simulink model "martin_arbot_v2offset"  (R2020a)
settings: Solver=ode15s  StartTime=0.0  StopTime=15  MaxStep=.01  RelTol=1e-3  AbsTol=1e-4
InitFcn:
  | % currentFolder = pwd;
  | % parent = '../Targeting';
  | % environment = '../Environment';
  | % addpath(genpath(parent));
  | % addpath(genpath(environment));
  | 
  | startup_ARbot;
  | chute2_DataFile;
  | guard_DataFile1;
  | shelf_DataFile1;
  | bin_assembly_DataFile;
values from neighbouring files (symbols this model uses):
  Environment = append(cwd,'/Environment')    [init_root_paths_mac.m]    (also in init_root_paths_windows.m = append(cwd,'\Environment'))
undefined symbols (not defined in the file or in its folder): belt_h, belt_l, belt_spd, belt_w, box1_dim, box2_dim, box3_dim, box4_dim, box5_dim, cube_d, deposit_joint_angle, Extr_Data_LinkHoles, floor_d, floor_l, ikSol, initial_joints, m, n, P_C, safe_via_angles, sigbuilder_block, smiData, X, Y, Z
libraries: sm_lib x145, nesl_utility x78, Contact_Forces_Lib x10, simulink x5, Parts_Lib x5, dspsrcs4 x1
(part 4 of 5)

== system martin_arbot_v2offset/Bin//guard//shelf1/guard_1_RIGID2 ==
  ReferenceFrame : sm_lib/Frames and Transforms/Reference Frame
  Solid : sm_lib/Body Elements/File Solid  ExtGeomFileName=/Users/mcontr/repos/ARbot_Simulink/v3/Environment/meshes/guard_Default_sldprt.STEP  UnitType=FromFile  ExtGeomFileUnits=m  StepReaderType=HEX  ExportConvexHullGeometry=off  InertiaType=Custom  Mass=smiData.Solid(1).mass  MassUnits=kg  CenterOfMass=smiData.Solid(1).CoM  CenterOfMassUnits=in  MomentsOfInertia=smiData.Solid(1).MoI  MomentsOfInertiaUnits=kg*in^2  ProductsOfInertia=smiData.Solid(1).PoI  ProductsOfInertiaUnits=kg*in^2  BasedOnType=DensityFromFile  Density=1000  DensityUnits=kg/m^3  DoExposeReferenceFrame=on  SerializedFrames=<Frames/>  GraphicType=FromGeometry  MarkerShape=Sphere  MarkerSize=10  GraphicVisPropType=SimpleVisualProperties  GraphicDiffuseColor=smiData.Solid(1).color  GraphicSpecularColor=[0.5 0.5 0.5 1.0]  GraphicAmbientColor=[0.15 0.15 0.15 1.0]  GraphicEmissiveColor=[0.0 0.0 0.0 1.0]  GraphicShininess=75  GraphicOpacity=smiData.Solid(1).opacity
  F : PMIOPort  Side=Left
  connections:
  ReferenceFrame/RConn1 -- Solid/RConn1 -- F/RConn1

== system martin_arbot_v2offset/Bin//guard//shelf1/guard_1_RIGID3 ==
  ReferenceFrame : sm_lib/Frames and Transforms/Reference Frame
  Solid : sm_lib/Body Elements/File Solid  ExtGeomFileName=/Users/mcontr/repos/ARbot_Simulink/v3/Environment/meshes/guard_Default_sldprt.STEP  UnitType=FromFile  ExtGeomFileUnits=m  StepReaderType=HEX  ExportConvexHullGeometry=off  InertiaType=Custom  Mass=smiData.Solid(1).mass  MassUnits=kg  CenterOfMass=smiData.Solid(1).CoM  CenterOfMassUnits=in  MomentsOfInertia=smiData.Solid(1).MoI  MomentsOfInertiaUnits=kg*in^2  ProductsOfInertia=smiData.Solid(1).PoI  ProductsOfInertiaUnits=kg*in^2  BasedOnType=DensityFromFile  Density=1000  DensityUnits=kg/m^3  DoExposeReferenceFrame=on  SerializedFrames=<Frames/>  GraphicType=FromGeometry  MarkerShape=Sphere  MarkerSize=10  GraphicVisPropType=SimpleVisualProperties  GraphicDiffuseColor=smiData.Solid(1).color  GraphicSpecularColor=[0.5 0.5 0.5 1.0]  GraphicAmbientColor=[0.15 0.15 0.15 1.0]  GraphicEmissiveColor=[0.0 0.0 0.0 1.0]  GraphicShininess=75  GraphicOpacity=smiData.Solid(1).opacity
  F : PMIOPort  Side=Left
  connections:
  ReferenceFrame/RConn1 -- Solid/RConn1 -- F/RConn1

== system martin_arbot_v2offset/Bin//guard//shelf1/shelf_1_RIGID1 ==
  ReferenceFrame : sm_lib/Frames and Transforms/Reference Frame
  Solid : sm_lib/Body Elements/File Solid  ExtGeomFileName=/Users/mcontr/repos/ARbot_Simulink/v3/Environment/meshes/shelf_Default_sldprt.STEP  UnitType=FromFile  ExtGeomFileUnits=m  StepReaderType=HEX  ExportConvexHullGeometry=off  InertiaType=Custom  Mass=smiData.Solid(1).mass  MassUnits=kg  CenterOfMass=smiData.Solid(1).CoM  CenterOfMassUnits=in  MomentsOfInertia=smiData.Solid(1).MoI  MomentsOfInertiaUnits=kg*in^2  ProductsOfInertia=smiData.Solid(1).PoI  ProductsOfInertiaUnits=kg*in^2  BasedOnType=DensityFromFile  Density=1000  DensityUnits=kg/m^3  DoExposeReferenceFrame=on  SerializedFrames=<Frames/>  GraphicType=FromGeometry  MarkerShape=Sphere  MarkerSize=10  GraphicVisPropType=SimpleVisualProperties  GraphicDiffuseColor=smiData.Solid(1).color  GraphicSpecularColor=[0.5 0.5 0.5 1.0]  GraphicAmbientColor=[0.15 0.15 0.15 1.0]  GraphicEmissiveColor=[0.0 0.0 0.0 1.0]  GraphicShininess=75  GraphicOpacity=smiData.Solid(1).opacity
  F : PMIOPort  Side=Left
  connections:
  ReferenceFrame/RConn1 -- Solid/RConn1 -- F/RConn1

== system martin_arbot_v2offset/Box1/Box1 ==
  Box : sm_lib/Body Elements/Brick Solid  GraphicAmbientColor=[0.15 0.15 0.15 1.0]  BasedOnType=Density  BrickDimensions=box1_dim  BrickDimensionUnits=m  CenterOfMass=[0 0 0]  CenterOfMassUnits=m  GraphicDiffuseColor=[0.7 0.3 .08]  Density=1000  DensityUnits=kg/m^3  DoExposeReferenceFrame=on  GraphicEmissiveColor=[0.0 0.0 0.0 1.0]  ExportEntireGeometry=off  SerializedFrames=<Frames/>  MarkerShape=Sphere  MarkerSize=10  GraphicType=FromGeometry  InertiaType=CalculateFromGeometry  Mass=1  MassUnits=kg  MomentsOfInertia=[1 1 1]  MomentsOfInertiaUnits=kg*m^2  GraphicOpacity=1.0  ProductsOfInertia=[1 1 1]  ProductsOfInertiaUnits=kg*m^2  GraphicShininess=75  GraphicSpecularColor=[0.5 0.5 0.5 1.0]  GraphicVisPropType=SimpleVisualProperties
  Transform Face px : sm_lib/Frames and Transforms/Rigid Transform  TranslationMethod=Cartesian  TranslationStandardOffset=0  TranslationLengthUnit=m  TranslationStandardAxis=+Z  TranslationCartesianOffset=[0 0 -box1_dim(3)*.5]  TranslationROffset=0  TranslationROffsetUnits=m  TranslationZOffset=0  TranslationZOffsetUnits=m  TranslationThetaOffset=0  TranslationThetaOffsetUnits=deg  RotationMethod=StandardAxis  RotationAngleUnits=deg  RotationStandardAxis=+X  RotationAngle=-180  RotationArbitraryAxis=[0 0 1]  FollAlignAxisA=+X  BaseAlignAxisA=+Y  FollAlignAxisB=+Y  BaseAlignAxisB=+Z  RotationSequenceAxes=FollowerAxes  RotationSequence=XYX  RotationSequenceAngles=[0 0 0]  RotationSequenceAnglesUnits=deg  RotationMatrix=[1 0 0; 0 1 0; 0 0 1]
  Fa : PMIOPort  Side=Right
  F : PMIOPort  Port=2  Side=Left
  connections:
  Fa/RConn1 -- Transform Face px/RConn1
  Transform Face px/LConn1 -- F/RConn1 -- Box/RConn1

== system martin_arbot_v2offset/Box1/Create Bus Belt In5 ==
  On : Inport
  Belt Speed : Gain  Gain=belt_spd
  Bus Creator : BusCreator  Inputs=3
  Constant : Constant
  Constant1 : Constant  Value=0
  bus : Outport  VectorParamsAs1DForOutWhenUnconnected=off
  wires:
  Constant1/1 -> Bus Creator/3  "vy"
  On/1 -> Belt Speed/1
  Constant/1 -> Bus Creator/1  "Enable"
  Bus Creator/1 -> bus/1
  Belt Speed/1 -> Bus Creator/2  "vx"

== system martin_arbot_v2offset/Box1/Forces5 ==
  B1 : Inport
  Bus Selector : BusSelector  OutputSignals=fz1.Normal Force,fz2.Normal Force,fz3.Normal Force,fz4.Normal Force
  Mux : Mux
  Fn1 : Outport  VectorParamsAs1DForOutWhenUnconnected=off
  wires:
  B1/1 -> Bus Selector/1
  Bus Selector/3 -> Mux/3  "<Normal Force>"
  Bus Selector/4 -> Mux/4  "<Normal Force>"
  Bus Selector/2 -> Mux/2  "<Normal Force>"
  Bus Selector/1 -> Mux/1  "<Normal Force>"
  Mux/1 -> Fn1/1

== system martin_arbot_v2offset/Box2/Box2 ==
  Box : sm_lib/Body Elements/Brick Solid  GraphicAmbientColor=[0.15 0.15 0.15 1.0]  BasedOnType=Density  BrickDimensions=box2_dim  BrickDimensionUnits=m  CenterOfMass=[0 0 0]  CenterOfMassUnits=m  GraphicDiffuseColor=[0.4 0.2 0.3]  Density=1000  DensityUnits=kg/m^3  DoExposeReferenceFrame=on  GraphicEmissiveColor=[0.0 0.0 0.0 1.0]  ExportEntireGeometry=off  SerializedFrames=<Frames/>  MarkerShape=Sphere  MarkerSize=10  GraphicType=FromGeometry  InertiaType=CalculateFromGeometry  Mass=1  MassUnits=kg  MomentsOfInertia=[1 1 1]  MomentsOfInertiaUnits=kg*m^2  GraphicOpacity=1.0  ProductsOfInertia=[1 1 1]  ProductsOfInertiaUnits=kg*m^2  GraphicShininess=75  GraphicSpecularColor=[0.5 0.5 0.5 1.0]  GraphicVisPropType=SimpleVisualProperties
  Transform Face px : sm_lib/Frames and Transforms/Rigid Transform  TranslationMethod=Cartesian  TranslationStandardOffset=0  TranslationLengthUnit=m  TranslationStandardAxis=+Z  TranslationCartesianOffset=[0 0 -box2_dim(3)*.5]  TranslationROffset=0  TranslationROffsetUnits=m  TranslationZOffset=0  TranslationZOffsetUnits=m  TranslationThetaOffset=0  TranslationThetaOffsetUnits=deg  RotationMethod=StandardAxis  RotationAngleUnits=deg  RotationStandardAxis=+X  RotationAngle=-180  RotationArbitraryAxis=[0 0 1]  FollAlignAxisA=+X  BaseAlignAxisA=+Y  FollAlignAxisB=+Y  BaseAlignAxisB=+Z  RotationSequenceAxes=FollowerAxes  RotationSequence=XYX  RotationSequenceAngles=[0 0 0]  RotationSequenceAnglesUnits=deg  RotationMatrix=[1 0 0; 0 1 0; 0 0 1]
  Fa : PMIOPort  Side=Right
  F : PMIOPort  Port=2  Side=Left
  connections:
  Fa/RConn1 -- Transform Face px/RConn1
  Transform Face px/LConn1 -- F/RConn1 -- Box/RConn1

== system martin_arbot_v2offset/Box2/Create Bus Belt In4 ==
  On : Inport
  Belt Speed : Gain  Gain=belt_spd
  Bus Creator : BusCreator  Inputs=3
  Constant : Constant
  Constant1 : Constant  Value=0
  bus : Outport  VectorParamsAs1DForOutWhenUnconnected=off
  wires:
  Constant1/1 -> Bus Creator/3  "vy"
  On/1 -> Belt Speed/1
  Constant/1 -> Bus Creator/1  "Enable"
  Bus Creator/1 -> bus/1
  Belt Speed/1 -> Bus Creator/2  "vx"

== system martin_arbot_v2offset/Box2/Forces4 ==
  B1 : Inport
  Bus Selector : BusSelector  OutputSignals=fz1.Normal Force,fz2.Normal Force,fz3.Normal Force,fz4.Normal Force
  Mux : Mux
  Fn1 : Outport  VectorParamsAs1DForOutWhenUnconnected=off
  wires:
  B1/1 -> Bus Selector/1
  Bus Selector/3 -> Mux/3  "<Normal Force>"
  Bus Selector/4 -> Mux/4  "<Normal Force>"
  Bus Selector/2 -> Mux/2  "<Normal Force>"
  Bus Selector/1 -> Mux/1  "<Normal Force>"
  Mux/1 -> Fn1/1

== system martin_arbot_v2offset/Box3/Box3 ==
  Box : sm_lib/Body Elements/Brick Solid  GraphicAmbientColor=[0.15 0.15 0.15 1.0]  BasedOnType=Density  BrickDimensions=box3_dim  BrickDimensionUnits=m  CenterOfMass=[0 0 0]  CenterOfMassUnits=m  GraphicDiffuseColor=[0.2 0.2 1.0]  Density=1000  DensityUnits=kg/m^3  DoExposeReferenceFrame=on  GraphicEmissiveColor=[0.0 0.0 0.0 1.0]  ExportEntireGeometry=off  SerializedFrames=<Frames/>  MarkerShape=Sphere  MarkerSize=10  GraphicType=FromGeometry  InertiaType=CalculateFromGeometry  Mass=1  MassUnits=kg  MomentsOfInertia=[1 1 1]  MomentsOfInertiaUnits=kg*m^2  GraphicOpacity=1.0  ProductsOfInertia=[1 1 1]  ProductsOfInertiaUnits=kg*m^2  GraphicShininess=75  GraphicSpecularColor=[0.5 0.5 0.5 1.0]  GraphicVisPropType=SimpleVisualProperties
  Transform Face px : sm_lib/Frames and Transforms/Rigid Transform  TranslationMethod=Cartesian  TranslationStandardOffset=0  TranslationLengthUnit=m  TranslationStandardAxis=+Z  TranslationCartesianOffset=[0 0 -box3_dim(3)*.5]  TranslationROffset=0  TranslationROffsetUnits=m  TranslationZOffset=0  TranslationZOffsetUnits=m  TranslationThetaOffset=0  TranslationThetaOffsetUnits=deg  RotationMethod=StandardAxis  RotationAngleUnits=deg  RotationStandardAxis=+X  RotationAngle=-180  RotationArbitraryAxis=[0 0 1]  FollAlignAxisA=+X  BaseAlignAxisA=+Y  FollAlignAxisB=+Y  BaseAlignAxisB=+Z  RotationSequenceAxes=FollowerAxes  RotationSequence=XYX  RotationSequenceAngles=[0 0 0]  RotationSequenceAnglesUnits=deg  RotationMatrix=[1 0 0; 0 1 0; 0 0 1]
  Fa : PMIOPort  Side=Right
  F : PMIOPort  Port=2  Side=Left
  connections:
  Fa/RConn1 -- Transform Face px/RConn1
  Transform Face px/LConn1 -- F/RConn1 -- Box/RConn1

== system martin_arbot_v2offset/Box3/Create Bus Belt In3 ==
  On : Inport
  Belt Speed : Gain  Gain=belt_spd
  Bus Creator : BusCreator  Inputs=3
  Constant : Constant
  Constant1 : Constant  Value=0
  bus : Outport  VectorParamsAs1DForOutWhenUnconnected=off
  wires:
  Constant1/1 -> Bus Creator/3  "vy"
  On/1 -> Belt Speed/1
  Constant/1 -> Bus Creator/1  "Enable"
  Bus Creator/1 -> bus/1
  Belt Speed/1 -> Bus Creator/2  "vx"

== system martin_arbot_v2offset/Box3/Forces3 ==
  B1 : Inport
  Bus Selector : BusSelector  OutputSignals=fz1.Normal Force,fz2.Normal Force,fz3.Normal Force,fz4.Normal Force
  Mux : Mux
  Fn1 : Outport  VectorParamsAs1DForOutWhenUnconnected=off
  wires:
  B1/1 -> Bus Selector/1
  Bus Selector/3 -> Mux/3  "<Normal Force>"
  Bus Selector/4 -> Mux/4  "<Normal Force>"
  Bus Selector/2 -> Mux/2  "<Normal Force>"
  Bus Selector/1 -> Mux/1  "<Normal Force>"
  Mux/1 -> Fn1/1

== system martin_arbot_v2offset/Box4/Box4 ==
  Box : sm_lib/Body Elements/Brick Solid  GraphicAmbientColor=[0.15 0.15 0.15 1.0]  BasedOnType=Density  BrickDimensions=box4_dim  BrickDimensionUnits=m  CenterOfMass=[0 0 0]  CenterOfMassUnits=m  GraphicDiffuseColor=[0.4 0.8 0.2]  Density=1000  DensityUnits=kg/m^3  DoExposeReferenceFrame=on  GraphicEmissiveColor=[0.0 0.0 0.0 1.0]  ExportEntireGeometry=off  SerializedFrames=<Frames/>  MarkerShape=Sphere  MarkerSize=10  GraphicType=FromGeometry  InertiaType=CalculateFromGeometry  Mass=1  MassUnits=kg  MomentsOfInertia=[1 1 1]  MomentsOfInertiaUnits=kg*m^2  GraphicOpacity=1.0  ProductsOfInertia=[1 1 1]  ProductsOfInertiaUnits=kg*m^2  GraphicShininess=75  GraphicSpecularColor=[0.5 0.5 0.5 1.0]  GraphicVisPropType=SimpleVisualProperties
  Transform Face px : sm_lib/Frames and Transforms/Rigid Transform  TranslationMethod=Cartesian  TranslationStandardOffset=0  TranslationLengthUnit=m  TranslationStandardAxis=+Z  TranslationCartesianOffset=[0 0 -box4_dim(3)*.5]  TranslationROffset=0  TranslationROffsetUnits=m  TranslationZOffset=0  TranslationZOffsetUnits=m  TranslationThetaOffset=0  TranslationThetaOffsetUnits=deg  RotationMethod=StandardAxis  RotationAngleUnits=deg  RotationStandardAxis=+X  RotationAngle=-180  RotationArbitraryAxis=[0 0 1]  FollAlignAxisA=+X  BaseAlignAxisA=+Y  FollAlignAxisB=+Y  BaseAlignAxisB=+Z  RotationSequenceAxes=FollowerAxes  RotationSequence=XYX  RotationSequenceAngles=[0 0 0]  RotationSequenceAnglesUnits=deg  RotationMatrix=[1 0 0; 0 1 0; 0 0 1]
  Fa : PMIOPort  Side=Right
  F : PMIOPort  Port=2  Side=Left
  connections:
  Fa/RConn1 -- Transform Face px/RConn1
  Transform Face px/LConn1 -- F/RConn1 -- Box/RConn1

== system martin_arbot_v2offset/Box4/Create Bus Belt In1 ==
  On : Inport
  Belt Speed : Gain  Gain=belt_spd
  Bus Creator : BusCreator  Inputs=3
  Constant : Constant
  Constant1 : Constant  Value=0
  bus : Outport  VectorParamsAs1DForOutWhenUnconnected=off
  wires:
  Constant1/1 -> Bus Creator/3  "vy"
  On/1 -> Belt Speed/1
  Constant/1 -> Bus Creator/1  "Enable"
  Bus Creator/1 -> bus/1
  Belt Speed/1 -> Bus Creator/2  "vx"

== system martin_arbot_v2offset/Box4/Forces1 ==
  B1 : Inport
  Bus Selector : BusSelector  OutputSignals=fz1.Normal Force,fz2.Normal Force,fz3.Normal Force,fz4.Normal Force
  Mux : Mux
  Fn1 : Outport  VectorParamsAs1DForOutWhenUnconnected=off
  wires:
  B1/1 -> Bus Selector/1
  Bus Selector/3 -> Mux/3  "<Normal Force>"
  Bus Selector/4 -> Mux/4  "<Normal Force>"
  Bus Selector/2 -> Mux/2  "<Normal Force>"
  Bus Selector/1 -> Mux/1  "<Normal Force>"
  Mux/1 -> Fn1/1

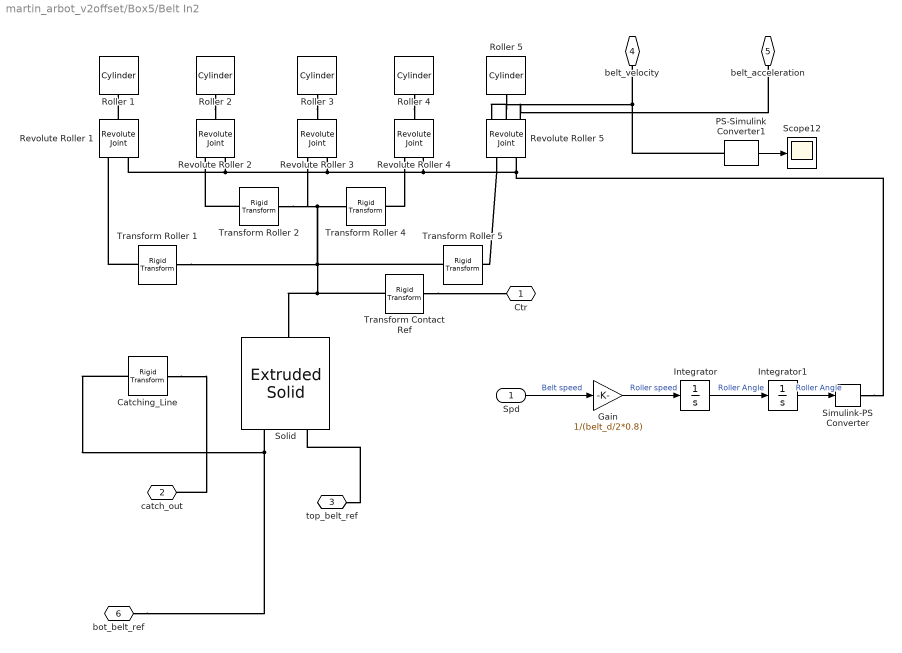
== system martin_arbot_v2offset/Box5/Belt In2 ==
  Spd : Inport
  Catching_Line : sm_lib/Frames and Transforms/Rigid Transform  TranslationMethod=StandardAxis  TranslationStandardOffset=catch_line_dist  TranslationLengthUnit=m  TranslationStandardAxis=+Y  TranslationCartesianOffset=[0 0 0]  TranslationROffset=0  TranslationROffsetUnits=m  TranslationZOffset=0  TranslationZOffsetUnits=m  TranslationThetaOffset=0  TranslationThetaOffsetUnits=deg  RotationMethod=StandardAxis  RotationAngleUnits=deg  RotationStandardAxis=+Y  RotationAngle=0.0  RotationArbitraryAxis=[0 0 1]  FollAlignAxisA=+X  BaseAlignAxisA=+Y  FollAlignAxisB=+Y  BaseAlignAxisB=+Z  RotationSequenceAxes=FollowerAxes  RotationSequence=XYX  RotationSequenceAngles=[0 0 0]  RotationSequenceAnglesUnits=deg  RotationMatrix=[1 0 0; 0 1 0; 0 0 1]
  Gain : Gain  Gain=1/(belt_d/2*0.8)
  Integrator : Integrator  InitialCondition=12.5049999999999
  Integrator1 : Integrator  InitialCondition=12.5049999999999
  PS-Simulink Converter1 : nesl_utility/PS-Simulink Converter  PhysicalDomain=network_engine_domain  SubClassName=ps_output  LeftPortType=input  RightPortType=output  PseudoPeriodic=off  Frequencies=[]  Unit=inherit  AffineConversion=off
  Revolute Roller {1..4} (4 alike) : sm_lib/Joints/Revolute Joint  JointMode=Normal  SenseConstraintForce=off  SenseConstraintForceX=off  SenseConstraintForceY=off  SenseConstraintForceZ=off  SenseConstraintTorque=off  SenseConstraintTorqueX=off  SenseConstraintTorqueY=off  SenseConstraintTorqueZ=off  SenseTotalForce=off  SenseTotalForceX=off  SenseTotalForceY=off  SenseTotalForceZ=off  SenseTotalTorque=off  SenseTotalTorqueX=off  SenseTotalTorqueY=off  SenseTotalTorqueZ=off  CompositeWrenchDir=FollowerOnBase  CompositeWrenchFrame=BaseFrame  EquilibriumPosition=0  EquilibriumPositionUnits=deg  SpringStiffness=0  SpringStiffnessUnits=N*m/deg  DampingCoefficient=0  DampingCoefficientUnits=N*m/(deg/s)  TorqueActuationMode=ComputedTorque  MotionActuationMode=InputMotion  SensePosition=off  SenseVelocity=off  SenseAcceleration=off  SenseTorqueForce=off  SenseLowerLimitTorqueForce=off  SenseUpperLimitTorqueForce=off  LowerLimitSpecify=off  LowerLimitBound=-90  LowerLimitBoundUnits=deg  LowerLimitStiffness=1e4  LowerLimitStiffnessUnits=N*m/deg  LowerLimitDamping=10  LowerLimitDampingUnits=N*m/(deg/s)  LowerLimitTransitionRegionWidth=0.1  LowerLimitTransitionRegionWidthUnits=deg  UpperLimitSpecify=off  UpperLimitBound=90  UpperLimitBoundUnits=deg  UpperLimitStiffness=1e4  UpperLimitStiffnessUnits=N*m/deg  UpperLimitDamping=10  UpperLimitDampingUnits=N*m/(deg/s)  UpperLimitTransitionRegionWidth=0.1  UpperLimitTransitionRegionWidthUnits=deg  PositionTargetSpecify=off  PositionTargetPriority=High  PositionTargetValue=0  PositionTargetValueUnits=deg  VelocityTargetSpecify=on  VelocityTargetPriority=High  VelocityTargetValue=12.5049999999992  VelocityTargetValueUnits=deg/s
  Revolute Roller 5 : sm_lib/Joints/Revolute Joint  JointMode=Normal  SenseConstraintForce=off  SenseConstraintForceX=off  SenseConstraintForceY=off  SenseConstraintForceZ=off  SenseConstraintTorque=off  SenseConstraintTorqueX=off  SenseConstraintTorqueY=off  SenseConstraintTorqueZ=off  SenseTotalForce=off  SenseTotalForceX=off  SenseTotalForceY=off  SenseTotalForceZ=off  SenseTotalTorque=off  SenseTotalTorqueX=off  SenseTotalTorqueY=off  SenseTotalTorqueZ=off  CompositeWrenchDir=FollowerOnBase  CompositeWrenchFrame=BaseFrame  EquilibriumPosition=0  EquilibriumPositionUnits=deg  SpringStiffness=0  SpringStiffnessUnits=N*m/deg  DampingCoefficient=0  DampingCoefficientUnits=N*m/(deg/s)  TorqueActuationMode=ComputedTorque  MotionActuationMode=InputMotion  SensePosition=off  SenseVelocity=on  SenseAcceleration=on  SenseTorqueForce=off  SenseLowerLimitTorqueForce=off  SenseUpperLimitTorqueForce=off  LowerLimitSpecify=off  LowerLimitBound=-90  LowerLimitBoundUnits=deg  LowerLimitStiffness=1e4  LowerLimitStiffnessUnits=N*m/deg  LowerLimitDamping=10  LowerLimitDampingUnits=N*m/(deg/s)  LowerLimitTransitionRegionWidth=0.1  LowerLimitTransitionRegionWidthUnits=deg  UpperLimitSpecify=off  UpperLimitBound=90  UpperLimitBoundUnits=deg  UpperLimitStiffness=1e4  UpperLimitStiffnessUnits=N*m/deg  UpperLimitDamping=10  UpperLimitDampingUnits=N*m/(deg/s)  UpperLimitTransitionRegionWidth=0.1  UpperLimitTransitionRegionWidthUnits=deg  PositionTargetSpecify=off  PositionTargetPriority=High  PositionTargetValue=0  PositionTargetValueUnits=deg  VelocityTargetSpecify=on  VelocityTargetPriority=High  VelocityTargetValue=12.5049999999992  VelocityTargetValueUnits=rad/s
  Roller {1..5} (5 alike) : Parts_Lib/Cylinder  Tag=CustomStyle  cyl_radius=belt_d/2*0.8  cyl_length=belt_w  cyl_density=1000  cyl_color=custom  cyl_opacity=1  cyl_color_custom=roller_clr  mark_radius=[0.75 0.5]  mark_len_factor=1.01  mark_angle=60  mark_color=black  mark_opacity=1
  Scope12 : Scope
  Simulink-PS Converter : nesl_utility/Simulink-PS Converter  PhysicalDomain=network_engine_domain  SubClassName=ps_input  LeftPortType=input  RightPortType=output  PseudoPeriodic=off  Frequencies=[]  NoiseDistribution=none  NoiseParameters=[]  Unit=1  AffineConversion=off  FilteringAndDerivatives=filter  SimscapeFilterOrder=2  InputFilterTimeConstant=0.005  UdotUserProvided=1
  Solid : sm_lib/Body Elements/Extruded Solid  GraphicAmbientColor=[0.15 0.15 0.15 1.0]  BasedOnType=Density  CenterOfMass=[0 0 0]  CenterOfMassUnits=m  GraphicDiffuseColor=[0.5 0.5 0.5]  ExportConvexHullGeometry=off  ExtrusionCrossSection=Extr_Data_LinkHoles(belt_l,belt_d,0.8*belt_d/2,5)  ExtrusionCrossSectionUnits=m  Density=1000  DensityUnits=kg/(m^3)  DoExposeReferenceFrame=on  GraphicEmissiveColor=[0.0 0.0 0.0 1.0]  ExportEntireGeometry=off  ExtrusionLength=belt_w  ExtrusionLengthUnits=m  ExtrusionType=General  SerializedFrames=<Frames><Frame><Id>Frame1</Id><Value><Name>camera_frame</Name><Origin><Source>GeometricFeature</Source><FeatureName>top point 723</FeatureName></Origin><PrimaryAxis><DefinedDirection>+Y</DefinedDirection><Source>ReferenceFrame</Source><SourceDirection>+X</SourceDirection><FeatureName></FeatureName></PrimaryAxis><SecondaryAxis><DefinedDirection>+X</DefinedDirection><Source>ReferenceFrame</Source><SourceDirection>-Z</SourceDirection><FeatureName></FeatureName></SecondaryAxis></Value></Frame><Frame><Id>Frame2</Id><Value><Name>End_Belt_Frame</Name><Origin><Source>GeometricFeature</Source><FeatureName>top point 2175</FeatureName></Origin><PrimaryAxis><DefinedDirection>+Z</DefinedDirection><Source>ReferenceFrame</Source><SourceDirection>+Y</SourceDirection><FeatureName></FeatureName></PrimaryAxis><SecondaryAxis><DefinedDirection>+Y</DefinedDirection><Source>ReferenceFrame</Source><SourceDirection>-X</SourceDirection><FeatureName></FeatureName></SecondaryAxis></Value></Frame></Frames>  MarkerShape=Sphere  MarkerSize=10  GraphicType=FromGeometry  InertiaType=CalculateFromGeometry  Mass=1  MassUnits=kg  MomentsOfInertia=[1 1 1]  MomentsOfInertiaUnits=kg*m^2  PolygonNumSides=3  GraphicOpacity=1.0  PolygonOuterRadius=1  PolygonOuterRadiusUnits=m  ProductsOfInertia=[0 0 0]  ProductsOfInertiaUnits=kg*m^2  GraphicShininess=75  GraphicSpecularColor=[0.5 0.5 0.5 1.0]  GraphicVisPropType=SimpleVisualProperties
  Transform Contact Ref : sm_lib/Frames and Transforms/Rigid Transform  TranslationMethod=None  TranslationStandardOffset=3/2  TranslationLengthUnit=m  TranslationStandardAxis=+X  TranslationCartesianOffset=[0 0 0]  TranslationROffset=0  TranslationROffsetUnits=m  TranslationZOffset=0  TranslationZOffsetUnits=m  TranslationThetaOffset=0  TranslationThetaOffsetUnits=deg  RotationMethod=RotationSequence  RotationAngleUnits=deg  RotationStandardAxis=+Z  RotationAngle=0  RotationArbitraryAxis=[0 0 1]  FollAlignAxisA=+X  BaseAlignAxisA=+Y  FollAlignAxisB=+Y  BaseAlignAxisB=+Z  RotationSequenceAxes=FollowerAxes  RotationSequence=XYZ  RotationSequenceAngles=[-90 0 0]  RotationSequenceAnglesUnits=deg  RotationMatrix=[1 0 0; 0 1 0; 0 0 1]
  Transform Roller 1 : sm_lib/Frames and Transforms/Rigid Transform  TranslationMethod=StandardAxis  TranslationStandardOffset=belt_l/2  TranslationLengthUnit=m  TranslationStandardAxis=-X  TranslationCartesianOffset=[0 0 0]  TranslationROffset=0  TranslationROffsetUnits=m  TranslationZOffset=0  TranslationZOffsetUnits=m  TranslationThetaOffset=0  TranslationThetaOffsetUnits=deg  RotationMethod=None  RotationAngleUnits=deg  RotationStandardAxis=+Z  RotationAngle=0  RotationArbitraryAxis=[0 0 1]  FollAlignAxisA=+X  BaseAlignAxisA=+Y  FollAlignAxisB=+Y  BaseAlignAxisB=+Z  RotationSequenceAxes=FollowerAxes  RotationSequence=XYX  RotationSequenceAngles=[0 0 0]  RotationSequenceAnglesUnits=deg  RotationMatrix=[1 0 0; 0 1 0; 0 0 1]
  Transform Roller 2 : sm_lib/Frames and Transforms/Rigid Transform  TranslationMethod=StandardAxis  TranslationStandardOffset=belt_l/4  TranslationLengthUnit=m  TranslationStandardAxis=-X  TranslationCartesianOffset=[0 0 0]  TranslationROffset=0  TranslationROffsetUnits=m  TranslationZOffset=0  TranslationZOffsetUnits=m  TranslationThetaOffset=0  TranslationThetaOffsetUnits=deg  RotationMethod=None  RotationAngleUnits=deg  RotationStandardAxis=+Z  RotationAngle=0  RotationArbitraryAxis=[0 0 1]  FollAlignAxisA=+X  BaseAlignAxisA=+Y  FollAlignAxisB=+Y  BaseAlignAxisB=+Z  RotationSequenceAxes=FollowerAxes  RotationSequence=XYX  RotationSequenceAngles=[0 0 0]  RotationSequenceAnglesUnits=deg  RotationMatrix=[1 0 0; 0 1 0; 0 0 1]
  Transform Roller 4 : sm_lib/Frames and Transforms/Rigid Transform  TranslationMethod=StandardAxis  TranslationStandardOffset=belt_l/4  TranslationLengthUnit=m  TranslationStandardAxis=+X  TranslationCartesianOffset=[0 0 0]  TranslationROffset=0  TranslationROffsetUnits=m  TranslationZOffset=0  TranslationZOffsetUnits=m  TranslationThetaOffset=0  TranslationThetaOffsetUnits=deg  RotationMethod=None  RotationAngleUnits=deg  RotationStandardAxis=+Z  RotationAngle=0  RotationArbitraryAxis=[0 0 1]  FollAlignAxisA=+X  BaseAlignAxisA=+Y  FollAlignAxisB=+Y  BaseAlignAxisB=+Z  RotationSequenceAxes=FollowerAxes  RotationSequence=XYX  RotationSequenceAngles=[0 0 0]  RotationSequenceAnglesUnits=deg  RotationMatrix=[1 0 0; 0 1 0; 0 0 1]
  Transform Roller 5 : sm_lib/Frames and Transforms/Rigid Transform  TranslationMethod=StandardAxis  TranslationStandardOffset=belt_l/2  TranslationLengthUnit=m  TranslationStandardAxis=+X  TranslationCartesianOffset=[0 0 0]  TranslationROffset=0  TranslationROffsetUnits=m  TranslationZOffset=0  TranslationZOffsetUnits=m  TranslationThetaOffset=0  TranslationThetaOffsetUnits=deg  RotationMethod=None  RotationAngleUnits=deg  RotationStandardAxis=+Z  RotationAngle=0  RotationArbitraryAxis=[0 0 1]  FollAlignAxisA=+X  BaseAlignAxisA=+Y  FollAlignAxisB=+Y  BaseAlignAxisB=+Z  RotationSequenceAxes=FollowerAxes  RotationSequence=XYX  RotationSequenceAngles=[0 0 0]  RotationSequenceAnglesUnits=deg  RotationMatrix=[1 0 0; 0 1 0; 0 0 1]
  Ctr : PMIOPort  Side=Right
  catch_out : PMIOPort  Port=2  Side=Left
  top_belt_ref : PMIOPort  Port=3  Side=Left
  belt_velocity : PMIOPort  Port=4  Side=Left
  belt_acceleration : PMIOPort  Port=5  Side=Left
  bot_belt_ref : PMIOPort  Port=6  Side=Left
  wires:
  Integrator/1 -> Integrator1/1  "Roller Angle"
  Gain/1 -> Integrator/1  "Roller speed"
  Spd/1 -> Gain/1  "Belt speed"
  PS-Simulink Converter1/1 -> Scope12/1
  Integrator1/1 -> Simulink-PS Converter/1  "Roller Angle"
  connections:
  Revolute Roller 5/LConn2 -- Revolute Roller 4/LConn2 -- Revolute Roller 3/LConn2 -- Revolute Roller 2/LConn2 -- Revolute Roller 1/LConn2 -- Simulink-PS Converter/RConn1
  Roller 5/LConn1 -- Revolute Roller 5/RConn1
  Roller 4/LConn1 -- Revolute Roller 4/RConn1
  Roller 3/LConn1 -- Revolute Roller 3/RConn1
  Roller 2/LConn1 -- Revolute Roller 2/RConn1
  Transform Roller 1/RConn1 -- Revolute Roller 1/LConn1
  Revolute Roller 5/LConn1 -- Transform Roller 5/RConn1
  Revolute Roller 4/LConn1 -- Transform Roller 4/RConn1
  Transform Roller 2/RConn1 -- Revolute Roller 2/LConn1
  Revolute Roller 1/RConn1 -- Roller 1/LConn1
  Transform Contact Ref/RConn1 -- Transform Roller 5/LConn1 -- Transform Roller 1/LConn1 -- Transform Roller 4/LConn1 -- Transform Roller 2/LConn1 -- Revolute Roller 3/LConn1 -- Solid/RConn1
  Transform Contact Ref/LConn1 -- Ctr/RConn1
  Catching_Line/LConn1 -- Solid/LConn1 -- bot_belt_ref/RConn1
  Catching_Line/RConn1 -- catch_out/RConn1
  top_belt_ref/RConn1 -- Solid/LConn2
  Revolute Roller 5/RConn2 -- PS-Simulink Converter1/LConn1 -- belt_velocity/RConn1
  Revolute Roller 5/RConn3 -- belt_acceleration/RConn1

== system martin_arbot_v2offset/Box5/Box5 ==
  Box : sm_lib/Body Elements/Brick Solid  GraphicAmbientColor=[0.15 0.15 0.15 1.0]  BasedOnType=Density  BrickDimensions=box5_dim  BrickDimensionUnits=m  CenterOfMass=[0 0 0]  CenterOfMassUnits=m  GraphicDiffuseColor=[0.8 0.2 .8]  Density=1000  DensityUnits=kg/m^3  DoExposeReferenceFrame=on  GraphicEmissiveColor=[0.0 0.0 0.0 1.0]  ExportEntireGeometry=off  SerializedFrames=<Frames/>  MarkerShape=Sphere  MarkerSize=10  GraphicType=FromGeometry  InertiaType=CalculateFromGeometry  Mass=1  MassUnits=kg  MomentsOfInertia=[1 1 1]  MomentsOfInertiaUnits=kg*m^2  GraphicOpacity=1.0  ProductsOfInertia=[1 1 1]  ProductsOfInertiaUnits=kg*m^2  GraphicShininess=75  GraphicSpecularColor=[0.5 0.5 0.5 1.0]  GraphicVisPropType=SimpleVisualProperties
  Transform Face px : sm_lib/Frames and Transforms/Rigid Transform  TranslationMethod=Cartesian  TranslationStandardOffset=0  TranslationLengthUnit=m  TranslationStandardAxis=+Z  TranslationCartesianOffset=[0 0 -box5_dim(3).*.5]  TranslationROffset=0  TranslationROffsetUnits=m  TranslationZOffset=0  TranslationZOffsetUnits=m  TranslationThetaOffset=0  TranslationThetaOffsetUnits=deg  RotationMethod=StandardAxis  RotationAngleUnits=deg  RotationStandardAxis=+X  RotationAngle=-180  RotationArbitraryAxis=[0 0 1]  FollAlignAxisA=+X  BaseAlignAxisA=+Y  FollAlignAxisB=+Y  BaseAlignAxisB=+Z  RotationSequenceAxes=FollowerAxes  RotationSequence=XYX  RotationSequenceAngles=[0 0 0]  RotationSequenceAnglesUnits=deg  RotationMatrix=[1 0 0; 0 1 0; 0 0 1]
  Fa : PMIOPort  Side=Right
  F : PMIOPort  Port=2  Side=Left
  connections:
  Fa/RConn1 -- Transform Face px/RConn1
  Transform Face px/LConn1 -- F/RConn1 -- Box/RConn1

== system martin_arbot_v2offset/Box5/Create Bus Belt In2 ==
  On : Inport
  Belt Speed : Gain  Gain=belt_spd
  Bus Creator : BusCreator  Inputs=3
  Constant : Constant
  Constant1 : Constant  Value=0
  bus : Outport  VectorParamsAs1DForOutWhenUnconnected=off
  wires:
  Constant1/1 -> Bus Creator/3  "vy"
  On/1 -> Belt Speed/1
  Constant/1 -> Bus Creator/1  "Enable"
  Bus Creator/1 -> bus/1
  Belt Speed/1 -> Bus Creator/2  "vx"

== system martin_arbot_v2offset/Box5/Forces2 ==
  B1 : Inport
  Bus Selector : BusSelector  OutputSignals=fz1.Normal Force,fz2.Normal Force,fz3.Normal Force,fz4.Normal Force
  Mux : Mux
  Fn1 : Outport  VectorParamsAs1DForOutWhenUnconnected=off
  wires:
  B1/1 -> Bus Selector/1
  Bus Selector/3 -> Mux/3  "<Normal Force>"
  Bus Selector/4 -> Mux/4  "<Normal Force>"
  Bus Selector/2 -> Mux/2  "<Normal Force>"
  Bus Selector/1 -> Mux/1  "<Normal Force>"
  Mux/1 -> Fn1/1

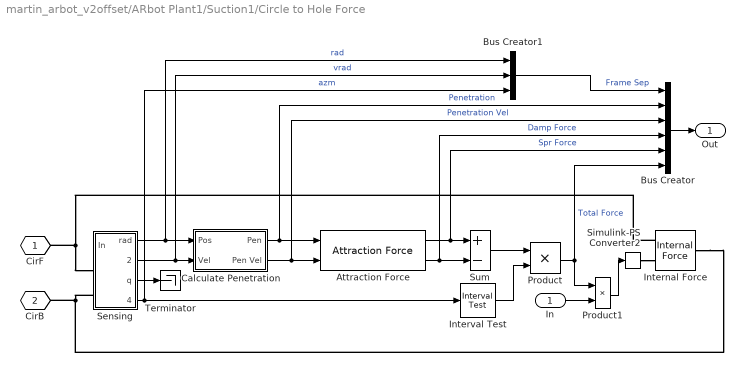
== system martin_arbot_v2offset/ARbot Plant1/Suction1/Circle to Hole Force ==
  In : Inport
  Attraction Force : Contact_Forces_Lib/Other Forces/Attraction Force  k_pen=k_contact  b_penvel=b_contact  max_sep=max_frame_sep  deadzone=h_deadzone
      settings: SourceProductName=Simscape Multibody Contact Forces Library
  Bus Creator : BusCreator  Inputs=6
  Bus Creator1 : BusCreator  Inputs=3
  Calculate Penetration : Subsystem
  Internal Force : sm_lib/Forces and Torques/Internal Force
      settings: SourceProductBaseCode=MS
  Interval Test : simulink/Logic and Bit Operations/Interval Test  IntervalClosedRight=on  uplimit=active_angle(2)  IntervalClosedLeft=on  lowlimit=active_angle(1)  OutDataTypeStr=uint8
  Product : Product
  Product1 : Product
  Sensing : Subsystem
  Simulink-PS Converter2 : nesl_utility/Simulink-PS Converter  PhysicalDomain=network_engine_domain  SubClassName=ps_input  LeftPortType=input  RightPortType=output  PseudoPeriodic=off  Frequencies=[]  NoiseDistribution=none  NoiseParameters=[]  Unit=1  AffineConversion=off  FilteringAndDerivatives=zero  SimscapeFilterOrder=1  InputFilterTimeConstant=0.005  UdotUserProvided=[]
  Sum : Sum  Inputs=+-
  Terminator : Terminator
  CirF : PMIOPort  Tag=PMCPort  Side=Left
  CirB : PMIOPort  Tag=PMCPort  Port=2  Side=Right
  Out : Outport  VectorParamsAs1DForOutWhenUnconnected=off
  wires:
  Bus Creator/1 -> Out/1
  Calculate Penetration/1(Pen) -> Bus Creator/2, Attraction Force/1  "Penetration"
  Bus Creator1/1 -> Bus Creator/1  "Frame Sep"
  Sensing/4(azm) -> Interval Test/1, Bus Creator1/3  "azm"
  Product/1 -> Product1/1, Bus Creator/6  "Total Force"
  Calculate Penetration/2(Pen Vel) -> Bus Creator/3, Attraction Force/2  "Penetration Vel"
  Sensing/2(vrad) -> Calculate Penetration/2(Vel), Bus Creator1/2  "vrad"
  Attraction Force/2 -> Sum/2, Bus Creator/4  "Damp Force"
  Sensing/1(rad) -> Calculate Penetration/1(Pos), Bus Creator1/1  "rad"
  Attraction Force/1 -> Sum/1, Bus Creator/5  "Spr Force"
  Sum/1 -> Product/1
  Sensing/3(q) -> Terminator/1
  Interval Test/1 -> Product/2
  In/1 -> Product1/2
  Product1/1 -> Simulink-PS Converter2/1
  connections:
  Simulink-PS Converter2/RConn1 -- Internal Force/LConn2
  CirF/RConn1 -- Sensing/LConn1 -- Internal Force/LConn1
  CirB/RConn1 -- Internal Force/RConn1 -- Sensing/LConn2

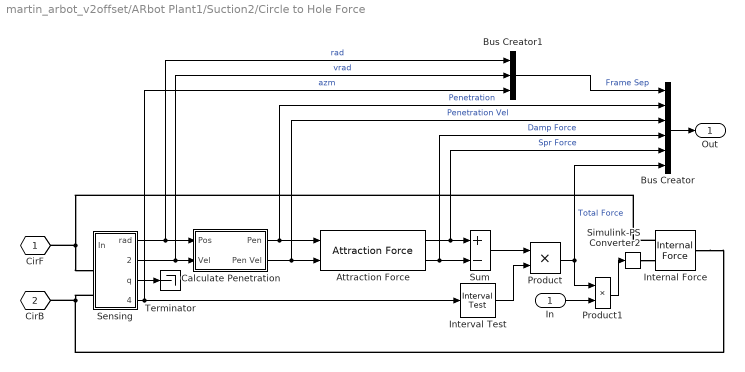
== system martin_arbot_v2offset/ARbot Plant1/Suction2/Circle to Hole Force ==
  In : Inport
  Attraction Force : Contact_Forces_Lib/Other Forces/Attraction Force  k_pen=k_contact  b_penvel=b_contact  max_sep=max_frame_sep  deadzone=h_deadzone
      settings: SourceProductName=Simscape Multibody Contact Forces Library
  Bus Creator : BusCreator  Inputs=6
  Bus Creator1 : BusCreator  Inputs=3
  Calculate Penetration : Subsystem
  Internal Force : sm_lib/Forces and Torques/Internal Force
      settings: SourceProductBaseCode=MS
  Interval Test : simulink/Logic and Bit Operations/Interval Test  IntervalClosedRight=on  uplimit=active_angle(2)  IntervalClosedLeft=on  lowlimit=active_angle(1)  OutDataTypeStr=uint8
  Product : Product
  Product1 : Product
  Sensing : Subsystem
  Simulink-PS Converter2 : nesl_utility/Simulink-PS Converter  PhysicalDomain=network_engine_domain  SubClassName=ps_input  LeftPortType=input  RightPortType=output  PseudoPeriodic=off  Frequencies=[]  NoiseDistribution=none  NoiseParameters=[]  Unit=1  AffineConversion=off  FilteringAndDerivatives=zero  SimscapeFilterOrder=1  InputFilterTimeConstant=0.005  UdotUserProvided=[]
  Sum : Sum  Inputs=+-
  Terminator : Terminator
  CirF : PMIOPort  Tag=PMCPort  Side=Left
  CirB : PMIOPort  Tag=PMCPort  Port=2  Side=Right
  Out : Outport  VectorParamsAs1DForOutWhenUnconnected=off
  wires:
  Product1/1 -> Simulink-PS Converter2/1
  In/1 -> Product1/2
  Interval Test/1 -> Product/2
  Sensing/3(q) -> Terminator/1
  Sum/1 -> Product/1
  Attraction Force/1 -> Bus Creator/5, Sum/1  "Spr Force"
  Sensing/1(rad) -> Bus Creator1/1, Calculate Penetration/1(Pos)  "rad"
  Attraction Force/2 -> Bus Creator/4, Sum/2  "Damp Force"
  Sensing/2(vrad) -> Bus Creator1/2, Calculate Penetration/2(Vel)  "vrad"
  Calculate Penetration/2(Pen Vel) -> Attraction Force/2, Bus Creator/3  "Penetration Vel"
  Product/1 -> Bus Creator/6, Product1/1  "Total Force"
  Sensing/4(azm) -> Bus Creator1/3, Interval Test/1  "azm"
  Bus Creator1/1 -> Bus Creator/1  "Frame Sep"
  Calculate Penetration/1(Pen) -> Attraction Force/1, Bus Creator/2  "Penetration"
  Bus Creator/1 -> Out/1
  connections:
  Sensing/LConn2 -- Internal Force/RConn1 -- CirB/RConn1
  Internal Force/LConn1 -- Sensing/LConn1 -- CirF/RConn1
  Simulink-PS Converter2/RConn1 -- Internal Force/LConn2

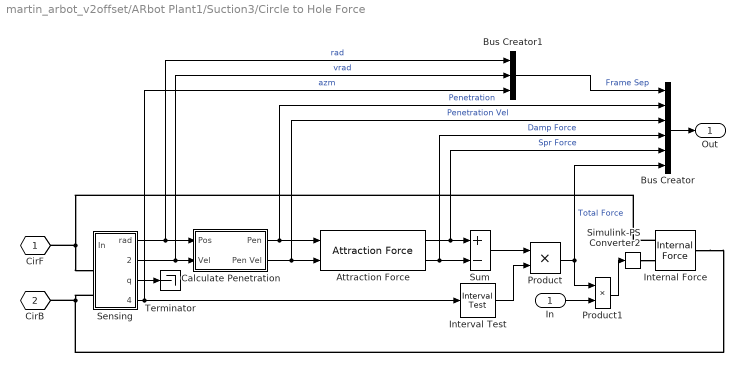
== system martin_arbot_v2offset/ARbot Plant1/Suction3/Circle to Hole Force ==
  In : Inport
  Attraction Force : Contact_Forces_Lib/Other Forces/Attraction Force  k_pen=k_contact  b_penvel=b_contact  max_sep=max_frame_sep  deadzone=h_deadzone
      settings: SourceProductName=Simscape Multibody Contact Forces Library
  Bus Creator : BusCreator  Inputs=6
  Bus Creator1 : BusCreator  Inputs=3
  Calculate Penetration : Subsystem
  Internal Force : sm_lib/Forces and Torques/Internal Force
      settings: SourceProductBaseCode=MS
  Interval Test : simulink/Logic and Bit Operations/Interval Test  IntervalClosedRight=on  uplimit=active_angle(2)  IntervalClosedLeft=on  lowlimit=active_angle(1)  OutDataTypeStr=uint8
  Product : Product
  Product1 : Product
  Sensing : Subsystem
  Simulink-PS Converter2 : nesl_utility/Simulink-PS Converter  PhysicalDomain=network_engine_domain  SubClassName=ps_input  LeftPortType=input  RightPortType=output  PseudoPeriodic=off  Frequencies=[]  NoiseDistribution=none  NoiseParameters=[]  Unit=1  AffineConversion=off  FilteringAndDerivatives=zero  SimscapeFilterOrder=1  InputFilterTimeConstant=0.005  UdotUserProvided=[]
  Sum : Sum  Inputs=+-
  Terminator : Terminator
  CirF : PMIOPort  Tag=PMCPort  Side=Left
  CirB : PMIOPort  Tag=PMCPort  Port=2  Side=Right
  Out : Outport  VectorParamsAs1DForOutWhenUnconnected=off
  wires:
  Bus Creator/1 -> Out/1
  Calculate Penetration/1(Pen) -> Bus Creator/2, Attraction Force/1  "Penetration"
  Bus Creator1/1 -> Bus Creator/1  "Frame Sep"
  Sensing/4(azm) -> Interval Test/1, Bus Creator1/3  "azm"
  Product/1 -> Product1/1, Bus Creator/6  "Total Force"
  Calculate Penetration/2(Pen Vel) -> Bus Creator/3, Attraction Force/2  "Penetration Vel"
  Sensing/2(vrad) -> Calculate Penetration/2(Vel), Bus Creator1/2  "vrad"
  Attraction Force/2 -> Sum/2, Bus Creator/4  "Damp Force"
  Sensing/1(rad) -> Calculate Penetration/1(Pos), Bus Creator1/1  "rad"
  Attraction Force/1 -> Sum/1, Bus Creator/5  "Spr Force"
  Sum/1 -> Product/1
  Sensing/3(q) -> Terminator/1
  Interval Test/1 -> Product/2
  In/1 -> Product1/2
  Product1/1 -> Simulink-PS Converter2/1
  connections:
  Simulink-PS Converter2/RConn1 -- Internal Force/LConn2
  CirF/RConn1 -- Sensing/LConn1 -- Internal Force/LConn1
  CirB/RConn1 -- Internal Force/RConn1 -- Sensing/LConn2

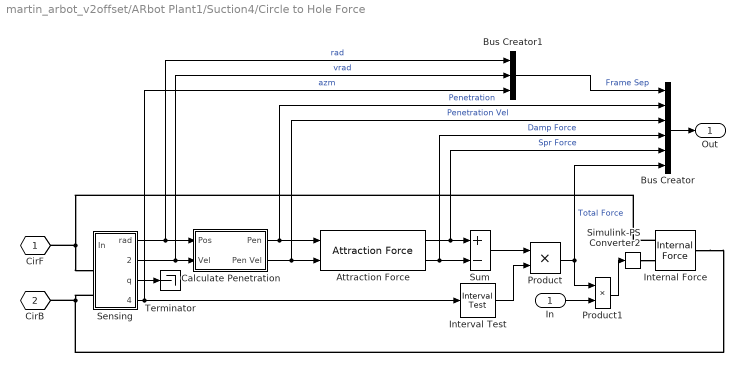
== system martin_arbot_v2offset/ARbot Plant1/Suction4/Circle to Hole Force ==
  In : Inport
  Attraction Force : Contact_Forces_Lib/Other Forces/Attraction Force  k_pen=k_contact  b_penvel=b_contact  max_sep=max_frame_sep  deadzone=h_deadzone
      settings: SourceProductName=Simscape Multibody Contact Forces Library
  Bus Creator : BusCreator  Inputs=6
  Bus Creator1 : BusCreator  Inputs=3
  Calculate Penetration : Subsystem
  Internal Force : sm_lib/Forces and Torques/Internal Force
      settings: SourceProductBaseCode=MS
  Interval Test : simulink/Logic and Bit Operations/Interval Test  IntervalClosedRight=on  uplimit=active_angle(2)  IntervalClosedLeft=on  lowlimit=active_angle(1)  OutDataTypeStr=uint8
  Product : Product
  Product1 : Product
  Sensing : Subsystem
  Simulink-PS Converter2 : nesl_utility/Simulink-PS Converter  PhysicalDomain=network_engine_domain  SubClassName=ps_input  LeftPortType=input  RightPortType=output  PseudoPeriodic=off  Frequencies=[]  NoiseDistribution=none  NoiseParameters=[]  Unit=1  AffineConversion=off  FilteringAndDerivatives=zero  SimscapeFilterOrder=1  InputFilterTimeConstant=0.005  UdotUserProvided=[]
  Sum : Sum  Inputs=+-
  Terminator : Terminator
  CirF : PMIOPort  Tag=PMCPort  Side=Left
  CirB : PMIOPort  Tag=PMCPort  Port=2  Side=Right
  Out : Outport  VectorParamsAs1DForOutWhenUnconnected=off
  wires:
  Product1/1 -> Simulink-PS Converter2/1
  In/1 -> Product1/2
  Interval Test/1 -> Product/2
  Sensing/3(q) -> Terminator/1
  Sum/1 -> Product/1
  Attraction Force/1 -> Bus Creator/5, Sum/1  "Spr Force"
  Sensing/1(rad) -> Bus Creator1/1, Calculate Penetration/1(Pos)  "rad"
  Attraction Force/2 -> Bus Creator/4, Sum/2  "Damp Force"
  Sensing/2(vrad) -> Bus Creator1/2, Calculate Penetration/2(Vel)  "vrad"
  Calculate Penetration/2(Pen Vel) -> Attraction Force/2, Bus Creator/3  "Penetration Vel"
  Product/1 -> Bus Creator/6, Product1/1  "Total Force"
  Sensing/4(azm) -> Bus Creator1/3, Interval Test/1  "azm"
  Bus Creator1/1 -> Bus Creator/1  "Frame Sep"
  Calculate Penetration/1(Pen) -> Attraction Force/1, Bus Creator/2  "Penetration"
  Bus Creator/1 -> Out/1
  connections:
  Sensing/LConn2 -- Internal Force/RConn1 -- CirB/RConn1
  Internal Force/LConn1 -- Sensing/LConn1 -- CirF/RConn1
  Simulink-PS Converter2/RConn1 -- Internal Force/LConn2

== system martin_arbot_v2offset/ARbot Plant1/Suction5/Circle to Hole Force ==
  In : Inport
  Attraction Force : Contact_Forces_Lib/Other Forces/Attraction Force  k_pen=k_contact  b_penvel=b_contact  max_sep=max_frame_sep  deadzone=h_deadzone
      settings: SourceProductName=Simscape Multibody Contact Forces Library
  Bus Creator : BusCreator  Inputs=6
  Bus Creator1 : BusCreator  Inputs=3
  Calculate Penetration : Subsystem
  Internal Force : sm_lib/Forces and Torques/Internal Force
      settings: SourceProductBaseCode=MS
  Interval Test : simulink/Logic and Bit Operations/Interval Test  IntervalClosedRight=on  uplimit=active_angle(2)  IntervalClosedLeft=on  lowlimit=active_angle(1)  OutDataTypeStr=uint8
  Product : Product
  Product1 : Product
  Sensing : Subsystem
  Simulink-PS Converter2 : nesl_utility/Simulink-PS Converter  PhysicalDomain=network_engine_domain  SubClassName=ps_input  LeftPortType=input  RightPortType=output  PseudoPeriodic=off  Frequencies=[]  NoiseDistribution=none  NoiseParameters=[]  Unit=1  AffineConversion=off  FilteringAndDerivatives=zero  SimscapeFilterOrder=1  InputFilterTimeConstant=0.005  UdotUserProvided=[]
  Sum : Sum  Inputs=+-
  Terminator : Terminator
  CirF : PMIOPort  Tag=PMCPort  Side=Left
  CirB : PMIOPort  Tag=PMCPort  Port=2  Side=Right
  Out : Outport  VectorParamsAs1DForOutWhenUnconnected=off
  wires:
  Bus Creator/1 -> Out/1
  Calculate Penetration/1(Pen) -> Bus Creator/2, Attraction Force/1  "Penetration"
  Bus Creator1/1 -> Bus Creator/1  "Frame Sep"
  Sensing/4(azm) -> Interval Test/1, Bus Creator1/3  "azm"
  Product/1 -> Product1/1, Bus Creator/6  "Total Force"
  Calculate Penetration/2(Pen Vel) -> Bus Creator/3, Attraction Force/2  "Penetration Vel"
  Sensing/2(vrad) -> Calculate Penetration/2(Vel), Bus Creator1/2  "vrad"
  Attraction Force/2 -> Sum/2, Bus Creator/4  "Damp Force"
  Sensing/1(rad) -> Calculate Penetration/1(Pos), Bus Creator1/1  "rad"
  Attraction Force/1 -> Sum/1, Bus Creator/5  "Spr Force"
  Sum/1 -> Product/1
  Sensing/3(q) -> Terminator/1
  Interval Test/1 -> Product/2
  In/1 -> Product1/2
  Product1/1 -> Simulink-PS Converter2/1
  connections:
  Simulink-PS Converter2/RConn1 -- Internal Force/LConn2
  CirF/RConn1 -- Sensing/LConn1 -- Internal Force/LConn1
  CirB/RConn1 -- Internal Force/RConn1 -- Sensing/LConn2

== system martin_arbot_v2offset/ARbot Plant1/Suction1/Circle to Hole Force/Calculate Penetration ==
  Pos : Inport
  Vel : Inport  Port=2
  Constant : Constant  Value=max_frame_sep
  Dead Zone Outside : DeadZone  LowerValue=-inf  UpperValue=0  SaturateOnIntegerOverflow=on
  Gain2 : Gain  Gain=-1
  Sum1 : Sum  Inputs=|-+
  Pen : Outport  VectorParamsAs1DForOutWhenUnconnected=off
  Pen Vel : Outport  Port=2  VectorParamsAs1DForOutWhenUnconnected=off
  wires:
  Vel/1 -> Gain2/1
  Gain2/1 -> Pen Vel/1
  Dead Zone Outside/1 -> Pen/1
  Constant/1 -> Sum1/2
  Sum1/1 -> Dead Zone Outside/1
  Pos/1 -> Sum1/1

== system martin_arbot_v2offset/ARbot Plant1/Suction1/Circle to Hole Force/Sensing ==
  In : Inport
  PS-Simulink Converter1 : nesl_utility/PS-Simulink Converter  PhysicalDomain=network_engine_domain  SubClassName=ps_output  LeftPortType=input  RightPortType=output  PseudoPeriodic=off  Frequencies=[]  Unit=deg  AffineConversion=off
  PS-Simulink Converter4 : nesl_utility/PS-Simulink Converter  PhysicalDomain=network_engine_domain  SubClassName=ps_output  LeftPortType=input  RightPortType=output  PseudoPeriodic=off  Frequencies=[]  Unit=1  AffineConversion=off
  PS-Simulink Converter5 : nesl_utility/PS-Simulink Converter  PhysicalDomain=network_engine_domain  SubClassName=ps_output  LeftPortType=input  RightPortType=output  PseudoPeriodic=off  Frequencies=[]  Unit=1  AffineConversion=off
  PS-Simulink Converter6 : nesl_utility/PS-Simulink Converter  PhysicalDomain=network_engine_domain  SubClassName=ps_output  LeftPortType=input  RightPortType=output  PseudoPeriodic=off  Frequencies=[]  Unit=1  AffineConversion=off
  Product : Product
  Selector : Selector  NumberOfDimensions=2  InputPortWidth=3  IndexOptions=Index vector (dialog),Index vector (dialog)  Indices=[1],[1,2]  OutputSizes=1,1
  Sign : Signum  ZeroCross=off
  Transform Sensor : sm_lib/Frames and Transforms/Transform Sensor  MeasurementFrame=NonRotatingBase  SenseAngle=off  SenseAxis=off  SenseAngle1=off  SenseAngle2=off  SenseAngle3=off  SenseQ=off  SenseR=off  SenseOmegaX=off  SenseOmegaY=off  SenseOmegaZ=off  SenseOmega1=off  SenseOmega2=off  SenseOmega3=off  SenseQDot=off  SenseRDot=off  SenseAlphaX=off  SenseAlphaY=off  SenseAlphaZ=off  SenseAlpha1=off  SenseAlpha2=off  SenseAlpha3=off  SenseQDDot=off  SenseRDDot=off  SenseX=off  SenseY=off  SenseZ=off  SenseRad=on  SenseAzim=on  SenseDist=off  SenseInc=off  SenseXDot=off  SenseYDot=off  SenseZDot=off  SenseRadDot=on  SenseAzimDot=off  SenseDistDot=off  SenseIncDot=off  SenseXDDot=off  SenseYDDot=off  SenseZDDot=off  SenseRadDDot=off  SenseAzimDDot=off  SenseDistDDot=off  SenseIncDDot=off
  Transform Sensor1 : sm_lib/Frames and Transforms/Transform Sensor  MeasurementFrame=World  SenseAngle=off  SenseAxis=off  SenseAngle1=off  SenseAngle2=off  SenseAngle3=off  SenseQ=off  SenseR=on  SenseOmegaX=off  SenseOmegaY=off  SenseOmegaZ=off  SenseOmega1=off  SenseOmega2=off  SenseOmega3=off  SenseQDot=off  SenseRDot=off  SenseAlphaX=off  SenseAlphaY=off  SenseAlphaZ=off  SenseAlpha1=off  SenseAlpha2=off  SenseAlpha3=off  SenseQDDot=off  SenseRDDot=off  SenseX=off  SenseY=off  SenseZ=off  SenseRad=off  SenseAzim=off  SenseDist=off  SenseInc=off  SenseXDot=off  SenseYDot=off  SenseZDot=off  SenseRadDot=off  SenseAzimDot=off  SenseDistDot=off  SenseIncDot=off  SenseXDDot=off  SenseYDDot=off  SenseZDDot=off  SenseRadDDot=off  SenseAzimDDot=off  SenseDistDDot=off  SenseIncDDot=off
  F : PMIOPort  Side=Left
  B : PMIOPort  Port=2  Side=Left
  rad : Outport  VectorParamsAs1DForOutWhenUnconnected=off
  vrad : Outport  Port=2  VectorParamsAs1DForOutWhenUnconnected=off
  q : Outport  Port=3  VectorParamsAs1DForOutWhenUnconnected=off
  azm : Outport  Port=4  VectorParamsAs1DForOutWhenUnconnected=off
  wires:
  PS-Simulink Converter6/1 -> Selector/1
  Selector/1 -> q/1
  PS-Simulink Converter1/1 -> azm/1
  PS-Simulink Converter5/1 -> Sign/1, rad/1
  In/1 -> Product/2
  Product/1 -> ?
  Sign/1 -> Product/1
  PS-Simulink Converter4/1 -> vrad/1
  connections:
  F/RConn1 -- Transform Sensor/RConn1 -- Transform Sensor1/RConn1
  Transform Sensor/LConn1 -- B/RConn1 -- Transform Sensor1/LConn1
  PS-Simulink Converter6/LConn1 -- Transform Sensor1/RConn2
  PS-Simulink Converter1/LConn1 -- Transform Sensor/RConn3
  PS-Simulink Converter5/LConn1 -- Transform Sensor/RConn2
  PS-Simulink Converter4/LConn1 -- Transform Sensor/RConn4

== system martin_arbot_v2offset/ARbot Plant1/Suction2/Circle to Hole Force/Calculate Penetration ==
  Pos : Inport
  Vel : Inport  Port=2
  Constant : Constant  Value=max_frame_sep
  Dead Zone Outside : DeadZone  LowerValue=-inf  UpperValue=0  SaturateOnIntegerOverflow=on
  Gain2 : Gain  Gain=-1
  Sum1 : Sum  Inputs=|-+
  Pen : Outport  VectorParamsAs1DForOutWhenUnconnected=off
  Pen Vel : Outport  Port=2  VectorParamsAs1DForOutWhenUnconnected=off
  wires:
  Pos/1 -> Sum1/1
  Sum1/1 -> Dead Zone Outside/1
  Constant/1 -> Sum1/2
  Dead Zone Outside/1 -> Pen/1
  Gain2/1 -> Pen Vel/1
  Vel/1 -> Gain2/1
